simulink model "FINAL_SIMULINK_MODEL"  (R2015a)
settings: Solver=ode3  StartTime=0.0  StopTime=20  RelTol=1e-3
libraries: simulink x5, fuzblock x2
settings Model: Creator=BML  LastModifiedBy=BML
settings SolverCC: AutoInsertRateTranBlk=on

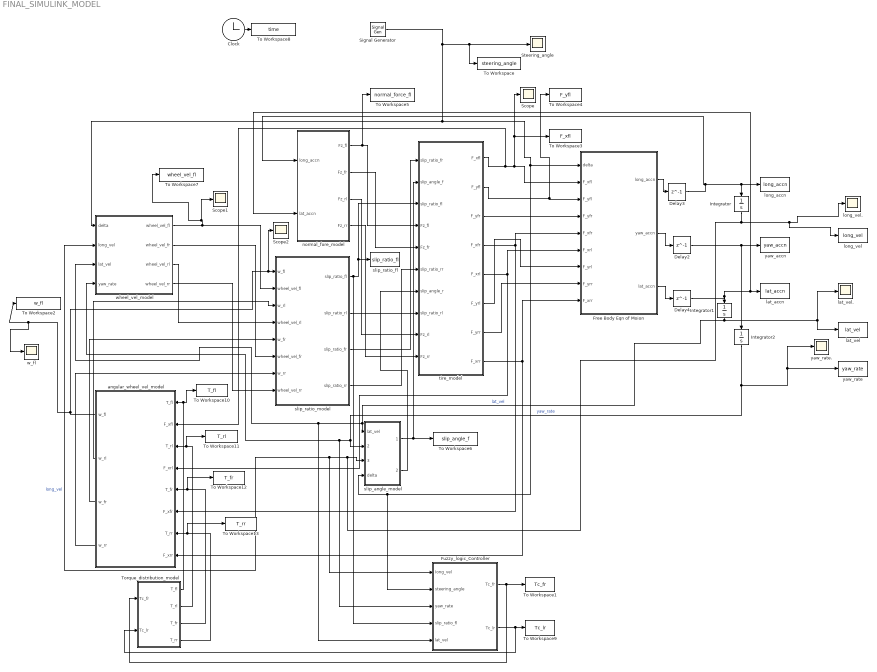
== system FINAL_SIMULINK_MODEL ==
  "           Steering_angle" : Scope
      settings: SaveName=ScopeData8
  Clock : Clock
  Delay2 : Delay  DelayLength=1  SampleTime=1
  Delay3 : Delay  DelayLength=1  SampleTime=1
  Delay4 : Delay  DelayLength=1  SampleTime=1
  Free Body Eqn of Moion : Subsystem
  Fuzzy_logic_Controller : Subsystem
  Integrator : Integrator  InitialCondition=22.22  LimitOutput=on  UpperSaturationLimit=23.22  LowerSaturationLimit=22.22
  Integrator1 : Integrator  LimitOutput=on  UpperSaturationLimit=10  LowerSaturationLimit=-10
  Integrator2 : Integrator  LimitOutput=on  UpperSaturationLimit=1  LowerSaturationLimit=-1
  Scope : Scope
      settings: SaveName=ScopeData3
  Scope1 : Scope
      settings: SaveName=ScopeData4
  Scope2 : Scope
      settings: SaveName=ScopeData6
  Signal Generator : SignalGenerator  Amplitude=2.5  Frequency=1.5  Units=rad/sec
  To Workspace : ToWorkspace  VariableName=steering_angle  SaveFormat=Timeseries  SampleTime=1
  To Workspace1 : ToWorkspace  VariableName=Tc_fr  SaveFormat=Timeseries  SampleTime=-1
  To Workspace10 : ToWorkspace  VariableName=T_fl  SaveFormat=Timeseries  SampleTime=1
  To Workspace11 : ToWorkspace  VariableName=T_rl  SaveFormat=Timeseries  SampleTime=1
  To Workspace12 : ToWorkspace  VariableName=T_fr  SaveFormat=Timeseries  SampleTime=1
  To Workspace13 : ToWorkspace  VariableName=T_rr  SaveFormat=Timeseries  SampleTime=1
  To Workspace2 : ToWorkspace  VariableName=w_fl  SaveFormat=Timeseries  SampleTime=1
  To Workspace3 : ToWorkspace  VariableName=F_xfl  SaveFormat=Timeseries  SampleTime=1
  To Workspace4 : ToWorkspace  VariableName=F_yfl  SaveFormat=Timeseries  SampleTime=1
  To Workspace5 : ToWorkspace  VariableName=normal_force_fl  SaveFormat=Timeseries  SampleTime=1
  To Workspace6 : ToWorkspace  VariableName=slip_angle_f  SaveFormat=Timeseries  SampleTime=1
  To Workspace7 : ToWorkspace  VariableName=wheel_vel_fl  SaveFormat=Timeseries  SampleTime=1
  To Workspace8 : ToWorkspace  VariableName=time  SaveFormat=Timeseries  SampleTime=1
  To Workspace9 : ToWorkspace  VariableName=Tc_lr  SaveFormat=Timeseries  SampleTime=-1
  Torque_distribution_model : Subsystem
  angular_wheel_vel_model : Subsystem
  lat_accn : ToWorkspace  VariableName=lat_accn  SaveFormat=Timeseries  SampleTime=1
  lat_vel : ToWorkspace  VariableName=lat_vel  SaveFormat=Timeseries  SampleTime=1
  lat_vel. : Scope
  long_accn : ToWorkspace  VariableName=long_accn  SaveFormat=Timeseries  SampleTime=1
  long_vel : ToWorkspace  VariableName=long_vel  SaveFormat=Timeseries  SampleTime=1
  long_vel. : Scope
  normal_fore_model : Subsystem
  slip_angle_model : Subsystem
  slip_ratio_fl : ToWorkspace  VariableName=slip_ratio_fl  SaveFormat=Timeseries  SampleTime=1
  slip_ratio_model : Subsystem
  tire_model : Subsystem
  w_fl : Scope
      settings: SaveName=ScopeData5
  wheel_vel_model : Subsystem
  yaw_accn : ToWorkspace  VariableName=yaw_accn  SaveFormat=Timeseries  SampleTime=1
  yaw_rate : ToWorkspace  VariableName=yaw_rate  SaveFormat=Timeseries  SampleTime=1
  yaw_rate. : Scope
      settings: SaveName=ScopeData2
  wires:
  slip_ratio_model/2(slip_ratio_rl) -> tire_model/8(slip_ratio_rl)
  Integrator2/1 -> slip_angle_model/2(yaw_rate), Fuzzy_logic_Controller/3(yaw_rate), wheel_vel_model/4(yaw_rate), yaw_rate./1, yaw_rate/1  "yaw_rate"
  normal_fore_model/1(Fz_fl) -> To Workspace5/1, tire_model/4(Fz_fl)
  normal_fore_model/2(Fz_fr) -> tire_model/5(Fz_fr)
  normal_fore_model/3(Fz_rl) -> tire_model/9(Fz_rl)
  normal_fore_model/4(Fz_rr) -> tire_model/10(Fz_rr)
  wheel_vel_model/3(wheel_vel_rl) -> slip_ratio_model/4(wheel_vel_rl)
  slip_ratio_model/3(slip_ratio_fr) -> tire_model/1(slip_ratio_fr)
  slip_ratio_model/4(slip_ratio_rr) -> tire_model/6(slip_ratio_rr)
  slip_angle_model/1(slip_angle_f) -> To Workspace6/1, tire_model/2("slip_angle_f  ")
  slip_angle_model/2(slip_angle_r) -> tire_model/7(slip_angle_r)
  wheel_vel_model/2(wheel_vel_fr) -> slip_ratio_model/6(wheel_vel_fr)
  wheel_vel_model/1(wheel_vel_fl) -> Scope1/1, To Workspace7/1, slip_ratio_model/2(wheel_vel_fl)
  wheel_vel_model/4(wheel_vel_rr) -> slip_ratio_model/8(wheel_vel_rr)
  Integrator/1 -> slip_angle_model/3(long_vel), Fuzzy_logic_Controller/1(Iong_vel), wheel_vel_model/2(long_vel), long_vel/1, long_vel./1  "long_vel"
  Integrator1/1 -> wheel_vel_model/3(lat_vel), Fuzzy_logic_Controller/5(lat_vel), slip_angle_model/1(lat_vel), lat_vel./1, lat_vel/1  "lat_vel"
  Free Body Eqn of Moion/2(yaw_accn) -> Delay2/1
  Free Body Eqn of Moion/1(long_accn) -> Delay3/1
  Free Body Eqn of Moion/3(lat_accn) -> Delay4/1
  angular_wheel_vel_model/4(w_rr) -> slip_ratio_model/7(w_rr)
  tire_model/3(F_yfr) -> Free Body Eqn of Moion/4(F_yfr)
  tire_model/6(F_yrl) -> Free Body Eqn of Moion/7(F_yrl)
  tire_model/7(F_yrr) -> Free Body Eqn of Moion/8(F_yrr)
  tire_model/2(F_yfl) -> To Workspace4/1, Free Body Eqn of Moion/3(F_yfl)
  Delay3/1 -> normal_fore_model/1(long_accn), Integrator/1, long_accn/1
  Delay4/1 -> normal_fore_model/2(lat_accn), lat_accn/1, Integrator1/1
  angular_wheel_vel_model/1(w_fl) -> Scope2/1, slip_ratio_model/1(w_fl), w_fl/1, To Workspace2/1
  angular_wheel_vel_model/2(w_rl) -> slip_ratio_model/3(w_rl)
  angular_wheel_vel_model/3(w_fr) -> slip_ratio_model/5(w_fr)
  Delay2/1 -> Integrator2/1, yaw_accn/1
  tire_model/1(F_xfl) -> angular_wheel_vel_model/2(F_xfl), Scope/1, To Workspace3/1, Free Body Eqn of Moion/2(F_xfl)
  tire_model/5(F_xrl) -> angular_wheel_vel_model/4(F_xrl), Free Body Eqn of Moion/6(F_xrl)
  tire_model/4(F_xfr) -> angular_wheel_vel_model/6(F_xfr), Free Body Eqn of Moion/5(F_xfr)
  tire_model/8(F_xrr) -> angular_wheel_vel_model/8(F_xrr), Free Body Eqn of Moion/9(F_xrr)
  Signal Generator/1 -> "           Steering_angle"/1, To Workspace/1, wheel_vel_model/1(delta), Fuzzy_logic_Controller/2(steering_angle), slip_angle_model/4(delta), Free Body Eqn of Moion/1(delta)
  slip_ratio_model/1(slip_ratio_fl) -> slip_ratio_fl/1, tire_model/3(slip_ratio_fl), Fuzzy_logic_Controller/4(slip_ratio_fl)
  Fuzzy_logic_Controller/1(Tc_fr) -> Torque_distribution_model/1(Tc_fr), To Workspace1/1
  Fuzzy_logic_Controller/2(Tc_lr) -> Torque_distribution_model/2(Tc_lr), To Workspace9/1
  Torque_distribution_model/1(T_fl) -> To Workspace10/1, angular_wheel_vel_model/1(T_fl)
  Torque_distribution_model/2(T_rl) -> To Workspace11/1, angular_wheel_vel_model/3(T_rl)
  Torque_distribution_model/3(T_fr) -> To Workspace12/1, angular_wheel_vel_model/5(T_fr)
  Torque_distribution_model/4(T_rr) -> To Workspace13/1, angular_wheel_vel_model/7(T_rr)
  Clock/1 -> To Workspace8/1

== system FINAL_SIMULINK_MODEL/Free Body Eqn of Moion ==
  delta : Inport
  F_xfl : Inport  Port=2
  F_yfl : Inport  Port=3
  F_yfr : Inport  Port=4
  F_xfr : Inport  Port=5
  F_xrl : Inport  Port=6
  F_yrl : Inport  Port=7
  F_yrr : Inport  Port=8
  F_xrr : Inport  Port=9
  lat_accn_model : Subsystem
  long_accn_model : Subsystem
  yaw_accn_model : Subsystem
  long_accn : Outport
  yaw_accn : Outport  Port=2
  lat_accn : Outport  Port=3
  wires:
  lat_accn_model/1(lat_accn) -> lat_accn/1
  F_yfl/1 -> long_accn_model/3(F_yfl), yaw_accn_model/3(F_yfl), lat_accn_model/3(F_yfl)
  delta/1 -> lat_accn_model/1(delta), yaw_accn_model/1(delta), long_accn_model/1(delta)
  F_xfr/1 -> long_accn_model/4(F_xfr), yaw_accn_model/4(F_xfr), lat_accn_model/4(F_xfr)
  F_yrl/1 -> yaw_accn_model/7(F_yrl), lat_accn_model/6(F_yrl)
  long_accn_model/1(long_accn) -> long_accn/1
  F_yfr/1 -> yaw_accn_model/5(F_yfr), long_accn_model/5(F_yfr), lat_accn_model/5(F_yfr)
  yaw_accn_model/1(yaw_accn) -> yaw_accn/1
  F_yrr/1 -> lat_accn_model/7(F_yrr), yaw_accn_model/9(F_yrr)
  F_xrl/1 -> long_accn_model/6(F_xrl), yaw_accn_model/6(F_xrl)
  F_xrr/1 -> long_accn_model/7(F_xrr), yaw_accn_model/8(F_xrr)
  F_xfl/1 -> long_accn_model/2(F_xfl), yaw_accn_model/2(F_xfl), lat_accn_model/2(F_xfl)

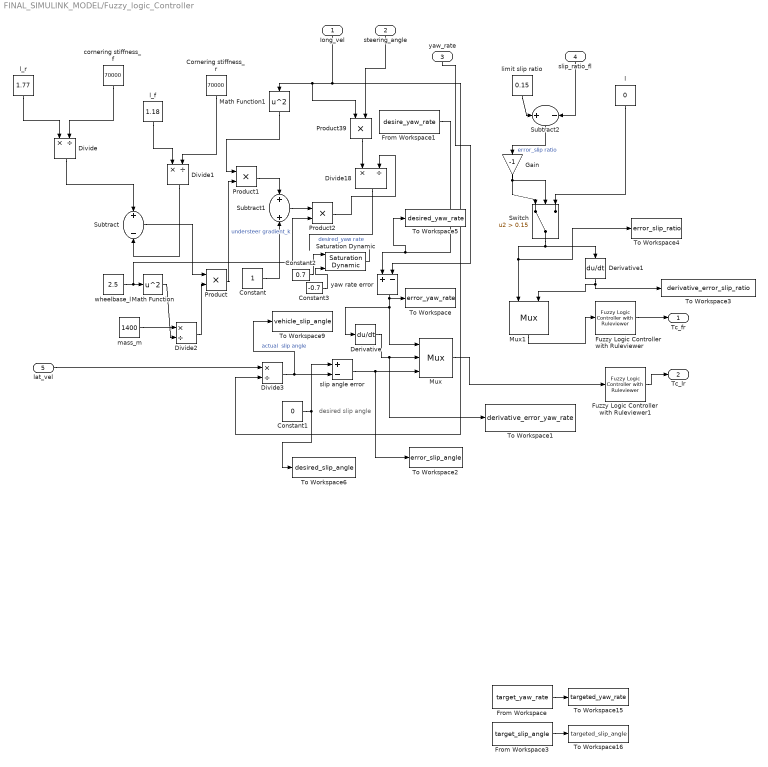
== system FINAL_SIMULINK_MODEL/Fuzzy_logic_Controller ==
  note: desired
      | slip angle
  Iong_vel : Inport
  steering_angle : Inport  Port=2
  yaw_rate : Inport  Port=3
  slip_ratio_fl : Inport  Port=4
  lat_vel : Inport  Port=5
  Constant : Constant
  Constant1 : Constant  Value=0
  Constant2 : Constant  Value=0.7
  Constant3 : Constant  Value=-0.7
  "Cornering stiffness_r " : Constant  Value=70000
  Derivative : Derivative
  Derivative1 : Derivative
  Divide{,1..3,18} (5 alike) : Product  Inputs=*/
  From Workspace : FromWorkspace  VariableName=target_yaw_rate  SampleTime=0
  From Workspace1 : FromWorkspace  VariableName=desire_yaw_rate  SampleTime=0
  From Workspace3 : FromWorkspace  VariableName=target_slip_angle  SampleTime=0
  Fuzzy Logic Controller with Ruleviewer : fuzblock/Fuzzy Logic  Controller  with Ruleviewer  fismatrix=fuzzy_slip_ratio1  Ts=2
  Fuzzy Logic Controller with Ruleviewer1 : fuzblock/Fuzzy Logic  Controller  with Ruleviewer  fismatrix=fuzzy_yaw_rate1  Ts=2
  Gain : Gain  Gain=-1
  Math Function : Math  Operator=square  SaturateOnIntegerOverflow=on
  Math Function1 : Math  Operator=square  SaturateOnIntegerOverflow=on
  Mux : Mux  Inputs=3
  Mux1 : Mux  Inputs=2
  Product{,1..2,39} (4 alike) : Product
  Saturation Dynamic : simulink/Discontinuities/Saturation Dynamic  OutMin=-0.7  OutMax=0.7  OutDataTypeStr=Inherit: Same as second input  OutDataType=fixdt(1, 16)  OutScaling=2^-10  DoSatur=off
  Subtract : Sum  Inputs=+-
  Subtract1 : Sum
  Subtract2 : Sum  Inputs=+-
  Switch : Switch  Criteria=u2 > Threshold  Threshold=0.15
  To Workspace : ToWorkspace  VariableName=error_yaw_rate  SaveFormat=Timeseries  SampleTime=1
  To Workspace1 : ToWorkspace  VariableName=derivative_error_yaw_rate  SaveFormat=Timeseries  SampleTime=1
  To Workspace15 : ToWorkspace  VariableName=targeted_yaw_rate  SaveFormat=Timeseries  SampleTime=1
  To Workspace16 : ToWorkspace  VariableName=targeted_slip_angle  SaveFormat=Timeseries  SampleTime=1
  To Workspace2 : ToWorkspace  VariableName=error_slip_angle  SaveFormat=Timeseries  SampleTime=1
  To Workspace3 : ToWorkspace  VariableName=derivative_error_slip_ratio  SaveFormat=Timeseries  SampleTime=1
  To Workspace4 : ToWorkspace  VariableName=error_slip_ratio  SaveFormat=Timeseries  SampleTime=1
  To Workspace5 : ToWorkspace  VariableName=desired_yaw_rate  SaveFormat=Timeseries  SampleTime=1
  To Workspace6 : ToWorkspace  VariableName=desired_slip_angle  SaveFormat=Timeseries  SampleTime=1
  To Workspace9 : ToWorkspace  VariableName=vehicle_slip_angle  SaveFormat=Timeseries  SampleTime=1
  "cornering stiffness_f " : Constant  Value=70000
  l : Constant  Value=0
  "l_f " : Constant  Value=1.18
  "l_r " : Constant  Value=1.77
  limit slip ratio : Constant  Value=0.15
  mass_m : Constant  Value=1400
  "slip angle error  " : Sum  Inputs=+-
  wheelbase_l : Constant  Value=2.5
  "yaw rate error   " : Sum  Inputs=+-
  Tc_fr : Outport
  Tc_lr : Outport  Port=2
  wires:
  Fuzzy Logic Controller with Ruleviewer/1 -> Tc_fr/1
  Divide/1 -> Subtract/1
  Subtract/1 -> Product/1
  Product/1 -> Product1/2  "understeer gradient_k"
  Constant/1 -> Subtract1/2
  Product39/1 -> Divide18/1
  Product2/1 -> Divide18/2
  steering_angle/1 -> Product39/2
  Math Function1/1 -> Product1/1
  Subtract1/1 -> Product2/1
  lat_vel/1 -> Divide3/1
  "l_r "/1 -> Divide/1
  Divide1/1 -> Subtract/2
  "Cornering stiffness_r "/1 -> Divide1/2
  wheelbase_l/1 -> Product2/2, Math Function/1
  mass_m/1 -> Divide2/1
  Math Function/1 -> Divide2/2
  Divide2/1 -> Product/2
  "l_f "/1 -> Divide1/1
  "cornering stiffness_f "/1 -> Divide/2
  Product1/1 -> Subtract1/1
  Switch/1 -> Mux1/1, To Workspace4/1, Derivative1/1
  yaw_rate/1 -> "yaw rate error   "/2
  Divide18/1 -> ?  "desired_yaw rate"
  Subtract2/1 -> Gain/1  "error_slip ratio"
  limit slip ratio/1 -> Subtract2/1
  Derivative/1 -> To Workspace1/1, Mux/2
  Mux/1 -> Fuzzy Logic Controller with Ruleviewer1/1
  slip_ratio_fl/1 -> Subtract2/2
  Divide3/1 -> To Workspace9/1, "slip angle error  "/2  "actual  slip angle"
  "slip angle error  "/1 -> To Workspace2/1, Mux/3
  Derivative1/1 -> Mux1/2, To Workspace3/1
  Mux1/1 -> Fuzzy Logic Controller with Ruleviewer/1
  Fuzzy Logic Controller with Ruleviewer1/1 -> Tc_lr/1
  "yaw rate error   "/1 -> To Workspace/1, Mux/1, Derivative/1
  Constant1/1 -> "slip angle error  "/1, To Workspace6/1
  Iong_vel/1 -> Divide3/2, Math Function1/1, Product39/1
  l/1 -> Switch/3
  Gain/1 -> Switch/1, Switch/2
  Constant2/1 -> Saturation Dynamic/1
  Constant3/1 -> Saturation Dynamic/3
  Saturation Dynamic/1 -> ?
  From Workspace1/1 -> To Workspace5/1, "yaw rate error   "/1
  From Workspace/1 -> To Workspace15/1
  From Workspace3/1 -> To Workspace16/1

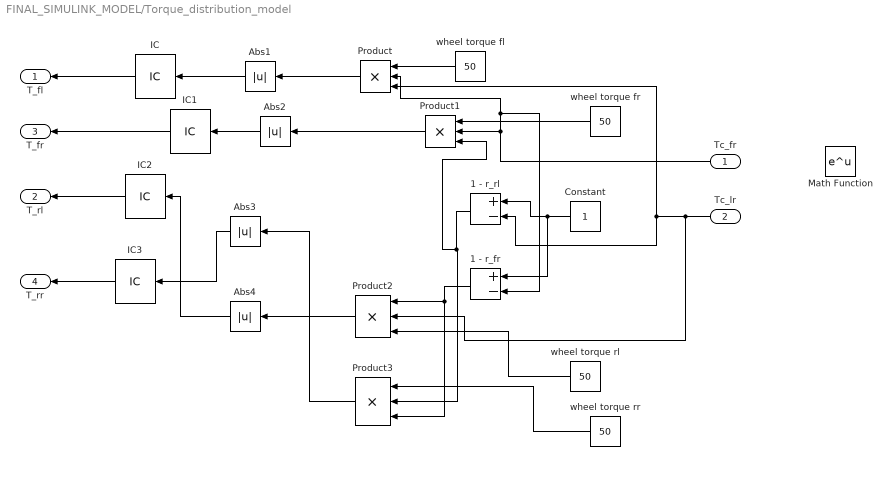
== system FINAL_SIMULINK_MODEL/Torque_distribution_model ==
  Tc_fr : Inport
  Tc_lr : Inport  Port=2
  1 - r_fr : Sum  Inputs=+-
  1 - r_rl : Sum  Inputs=+-
  Abs{1..4} (4 alike) : Abs
  Constant : Constant
  IC{,1..3} (4 alike) : InitialCondition  Value=50
  Math Function : Math  SaturateOnIntegerOverflow=on
  Product{,1..3} (4 alike) : Product  Inputs=3
  wheel torque fl : Constant  Value=50
  wheel torque fr : Constant  Value=50
  wheel torque rl : Constant  Value=50
  wheel torque rr : Constant  Value=50
  T_fl : Outport
  T_rl : Outport  Port=2
  T_fr : Outport  Port=3
  T_rr : Outport  Port=4
  wires:
  1 - r_rl/1 -> Product3/2, Product1/3
  Constant/1 -> 1 - r_fr/1, 1 - r_rl/1
  1 - r_fr/1 -> Product3/3, Product2/1
  wheel torque fl/1 -> Product/1
  Tc_fr/1 -> Product/2, 1 - r_fr/2, Product1/2
  Product1/1 -> Abs2/1
  Product3/1 -> Abs3/1
  Product2/1 -> Abs4/1
  Product/1 -> Abs1/1
  Tc_lr/1 -> Product2/2, 1 - r_rl/2, Product/3
  wheel torque fr/1 -> Product1/1
  wheel torque rl/1 -> Product2/3
  wheel torque rr/1 -> Product3/1
  Abs1/1 -> IC/1
  Abs2/1 -> IC1/1
  Abs3/1 -> IC3/1
  Abs4/1 -> IC2/1
  IC/1 -> T_fl/1
  IC1/1 -> T_fr/1
  IC2/1 -> T_rl/1
  IC3/1 -> T_rr/1

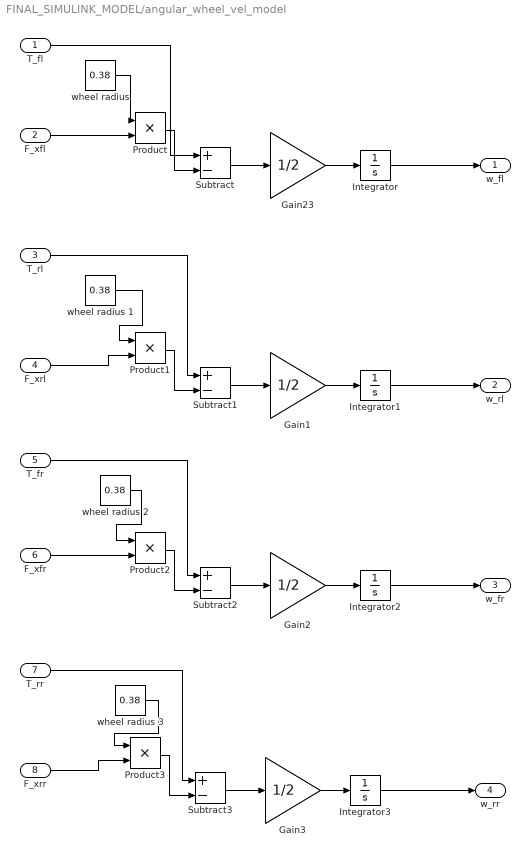
== system FINAL_SIMULINK_MODEL/angular_wheel_vel_model ==
  T_fl : Inport
  F_xfl : Inport  Port=2
  T_rl : Inport  Port=3
  F_xrl : Inport  Port=4
  T_fr : Inport  Port=5
  F_xfr : Inport  Port=6
  T_rr : Inport  Port=7
  F_xrr : Inport  Port=8
  Gain{1..3,23} (4 alike) : Gain  Gain=1/2
  Integrator{,1..3} (4 alike) : Integrator  InitialCondition=58.5  LimitOutput=on  UpperSaturationLimit=70  LowerSaturationLimit=57
  Product{,1..3} (4 alike) : Product
  Subtract{,1..3} (4 alike) : Sum  Inputs=+-
  wheel radius {,1..3} (4 alike) : Constant  Value=0.38
  w_fl : Outport
  w_rl : Outport  Port=2
  w_fr : Outport  Port=3
  w_rr : Outport  Port=4
  wires:
  Gain23/1 -> Integrator/1
  F_xfl/1 -> Product/2
  Product/1 -> Subtract/2
  wheel radius 1/1 -> Product1/1
  T_rl/1 -> Subtract1/1
  T_fl/1 -> Subtract/1
  Subtract/1 -> Gain23/1
  F_xrl/1 -> Product1/2
  "wheel radius "/1 -> Product/1
  Subtract2/1 -> Gain2/1
  wheel radius 2/1 -> Product2/1
  Product1/1 -> Subtract1/2
  F_xrr/1 -> Product3/2
  T_rr/1 -> Subtract3/1
  Gain3/1 -> Integrator3/1
  Subtract1/1 -> Gain1/1
  Gain1/1 -> Integrator1/1
  Gain2/1 -> Integrator2/1
  Subtract3/1 -> Gain3/1
  wheel radius 3/1 -> Product3/1
  F_xfr/1 -> Product2/2
  Product3/1 -> Subtract3/2
  T_fr/1 -> Subtract2/1
  Product2/1 -> Subtract2/2
  Integrator/1 -> w_fl/1
  Integrator1/1 -> w_rl/1
  Integrator2/1 -> w_fr/1
  Integrator3/1 -> w_rr/1

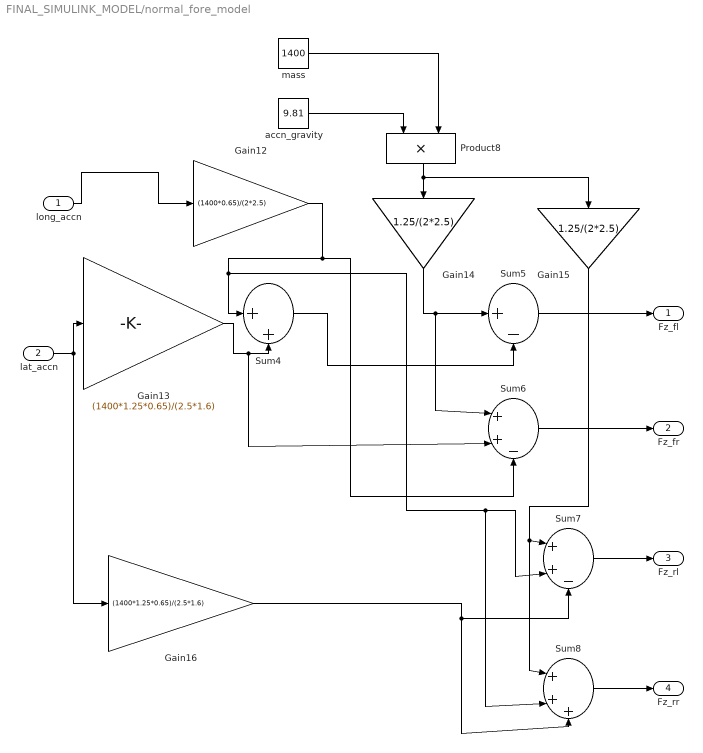
== system FINAL_SIMULINK_MODEL/normal_fore_model ==
  long_accn : Inport
  lat_accn : Inport  Port=2
  Gain12 : Gain  Gain=(1400*0.65)/(2*2.5)
  Gain13 : Gain  Gain=(1400*1.25*0.65)/(2.5*1.6)
  Gain14 : Gain  Gain=1.25/(2*2.5)
  Gain15 : Gain  Gain=1.25/(2*2.5)
  Gain16 : Gain  Gain=(1400*1.25*0.65)/(2.5*1.6)
  Product8 : Product
  Sum4 : Sum  Inputs=|++
  Sum5 : Sum  Inputs=|+-
  Sum6 : Sum  Inputs=|++-
  Sum7 : Sum  Inputs=|++-
  Sum8 : Sum  Inputs=|+++
  "accn_gravity " : Constant  Value=9.81
  mass : Constant  Value=1400
  Fz_fl : Outport
  Fz_fr : Outport  Port=2
  Fz_rl : Outport  Port=3
  Fz_rr : Outport  Port=4
  wires:
  Gain12/1 -> Sum4/1, Sum8/2, Sum7/2, Sum6/3
  Gain15/1 -> Sum8/1, Sum7/1
  Gain16/1 -> Sum8/3, Sum7/3
  Sum7/1 -> Fz_rl/1
  lat_accn/1 -> Gain13/1, Gain16/1
  Gain13/1 -> Sum6/2, Sum4/2
  Sum5/1 -> Fz_fl/1
  Sum6/1 -> Fz_fr/1
  Sum4/1 -> Sum5/2
  long_accn/1 -> Gain12/1
  mass/1 -> Product8/2
  Gain14/1 -> Sum5/1, Sum6/1
  Sum8/1 -> Fz_rr/1
  Product8/1 -> Gain14/1, Gain15/1
  "accn_gravity "/1 -> Product8/1

== system FINAL_SIMULINK_MODEL/slip_angle_model ==
  lat_vel : Inport
  yaw_rate : Inport  Port=2
  long_vel : Inport  Port=3
  delta : Inport  Port=4
  Divide4 : Product  Inputs=*/
  Divide5 : Product  Inputs=*/
  Product : Product
  Product1 : Product
  Sum4 : Sum  Inputs=|++
  Sum5 : Sum  Inputs=|+-
  Sum6 : Sum  Inputs=|+-
  l_f : Constant  Value=1.25
  l_r : Constant  Value=1.25
  slip_angle_f : Outport
  slip_angle_r : Outport  Port=2
  wires:
  yaw_rate/1 -> Product1/2, Product/2
  long_vel/1 -> Divide5/2, Divide4/2
  l_f/1 -> Product/1
  lat_vel/1 -> Sum6/2, Sum4/1
  Divide4/1 -> Sum5/2
  Product/1 -> Sum4/2
  Sum4/1 -> Divide4/1
  Divide5/1 -> slip_angle_r/1
  delta/1 -> Sum5/1
  Sum5/1 -> slip_angle_f/1
  Product1/1 -> Sum6/1
  l_r/1 -> Product1/1
  Sum6/1 -> Divide5/1

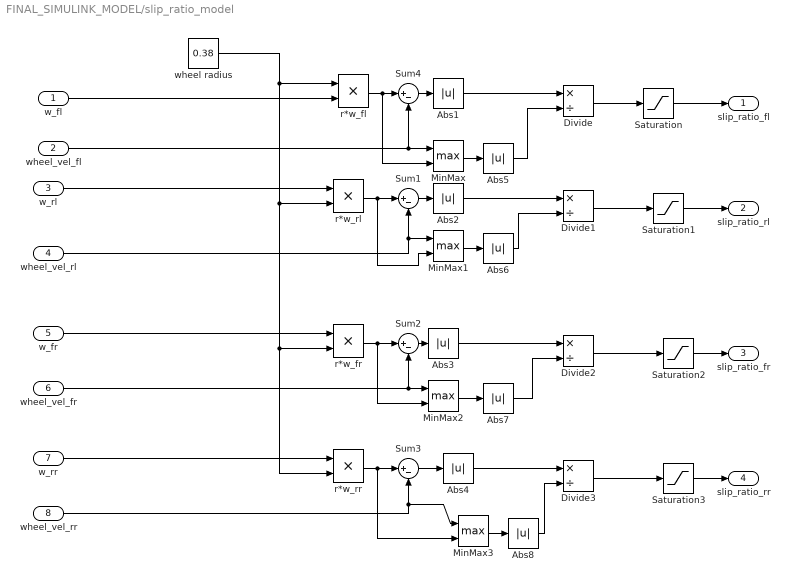
== system FINAL_SIMULINK_MODEL/slip_ratio_model ==
  w_fl : Inport
  wheel_vel_fl : Inport  Port=2
  w_rl : Inport  Port=3
  wheel_vel_rl : Inport  Port=4
  w_fr : Inport  Port=5
  wheel_vel_fr : Inport  Port=6
  w_rr : Inport  Port=7
  wheel_vel_rr : Inport  Port=8
  Abs{1..8} (8 alike) : Abs
  Divide{,1..3} (4 alike) : Product  Inputs=*/
  MinMax{,1..3} (4 alike) : MinMax  Function=max  Inputs=2
  Saturation{,1..3} (4 alike) : Saturate  UpperLimit=1  LowerLimit=0
  Sum{1..4} (4 alike) : Sum  Inputs=|+-
  r*w_fl : Product  Inputs=**
  r*w_fr : Product  Inputs=**
  r*w_rl : Product  Inputs=**
  r*w_rr : Product  Inputs=**
  wheel radius : Constant  Value=0.38
  slip_ratio_fl : Outport
  slip_ratio_rl : Outport  Port=2
  slip_ratio_fr : Outport  Port=3
  slip_ratio_rr : Outport  Port=4
  wires:
  w_fl/1 -> r*w_fl/2
  r*w_fl/1 -> MinMax/2, Sum4/1
  wheel radius/1 -> r*w_fl/1, r*w_rl/2, r*w_rr/2, r*w_fr/2
  wheel_vel_fl/1 -> MinMax/1, Sum4/2
  Sum4/1 -> Abs1/1
  Abs1/1 -> Divide/1
  MinMax/1 -> Abs5/1
  r*w_rl/1 -> MinMax1/2, Sum1/1
  wheel_vel_rl/1 -> Sum1/2, MinMax1/1
  Sum1/1 -> Abs2/1
  Abs2/1 -> Divide1/1
  MinMax1/1 -> Abs6/1
  w_rl/1 -> r*w_rl/1
  r*w_fr/1 -> MinMax2/2, Sum2/1
  wheel_vel_fr/1 -> Sum2/2, MinMax2/1
  Sum2/1 -> Abs3/1
  Abs3/1 -> Divide2/1
  MinMax2/1 -> Abs7/1
  w_fr/1 -> r*w_fr/1
  r*w_rr/1 -> MinMax3/2, Sum3/1
  wheel_vel_rr/1 -> MinMax3/1, Sum3/2
  Sum3/1 -> Abs4/1
  Abs4/1 -> Divide3/1
  MinMax3/1 -> Abs8/1
  w_rr/1 -> r*w_rr/1
  Divide/1 -> Saturation/1
  Divide1/1 -> Saturation1/1
  Divide2/1 -> Saturation2/1
  Divide3/1 -> Saturation3/1
  Abs5/1 -> Divide/2
  Abs6/1 -> Divide1/2
  Abs7/1 -> Divide2/2
  Abs8/1 -> Divide3/2
  Saturation/1 -> slip_ratio_fl/1
  Saturation1/1 -> slip_ratio_rl/1
  Saturation2/1 -> slip_ratio_fr/1
  Saturation3/1 -> slip_ratio_rr/1

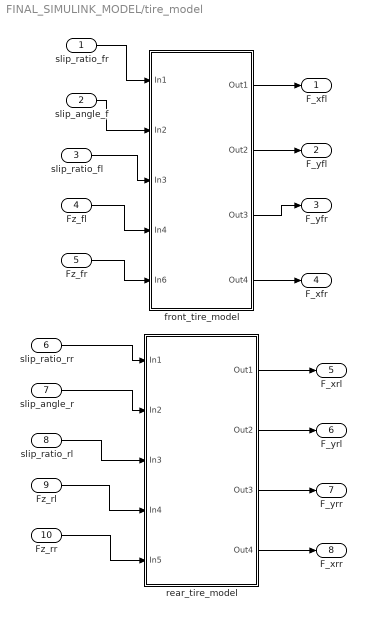
== system FINAL_SIMULINK_MODEL/tire_model ==
  slip_ratio_fr : Inport
  "slip_angle_f  " : Inport  Port=2
  slip_ratio_fl : Inport  Port=3
  Fz_fl : Inport  Port=4
  Fz_fr : Inport  Port=5
  slip_ratio_rr : Inport  Port=6
  slip_angle_r : Inport  Port=7
  slip_ratio_rl : Inport  Port=8
  Fz_rl : Inport  Port=9
  Fz_rr : Inport  Port=10
  front_tire_model : Subsystem
  rear_tire_model : Subsystem
  F_xfl : Outport
  F_yfl : Outport  Port=2
  F_yfr : Outport  Port=3
  F_xfr : Outport  Port=4
  F_xrl : Outport  Port=5
  F_yrl : Outport  Port=6
  F_yrr : Outport  Port=7
  F_xrr : Outport  Port=8
  wires:
  slip_ratio_rr/1 -> rear_tire_model/1(In1)
  slip_angle_r/1 -> rear_tire_model/2(In2)
  rear_tire_model/3(Out3) -> F_yrr/1
  slip_ratio_rl/1 -> rear_tire_model/3(In3)
  rear_tire_model/2(Out2) -> F_yrl/1
  Fz_rr/1 -> rear_tire_model/5(In5)
  rear_tire_model/1(Out1) -> F_xrl/1
  rear_tire_model/4(Out4) -> F_xrr/1
  Fz_rl/1 -> rear_tire_model/4(In4)
  "slip_angle_f  "/1 -> front_tire_model/2(In2)
  slip_ratio_fr/1 -> front_tire_model/1(In1)
  slip_ratio_fl/1 -> front_tire_model/3(In3)
  Fz_fr/1 -> front_tire_model/5(In6)
  front_tire_model/1(Out1) -> F_xfl/1
  front_tire_model/3(Out3) -> F_yfr/1
  front_tire_model/2(Out2) -> F_yfl/1
  Fz_fl/1 -> front_tire_model/4(In4)
  front_tire_model/4(Out4) -> F_xfr/1

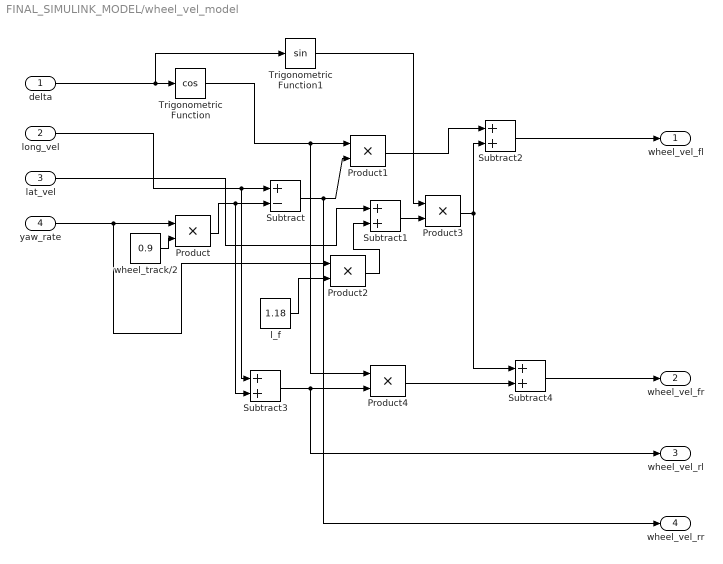
== system FINAL_SIMULINK_MODEL/wheel_vel_model ==
  delta : Inport
  long_vel : Inport  Port=2
  lat_vel : Inport  Port=3
  yaw_rate : Inport  Port=4
  Product{,1..4} (5 alike) : Product
  Subtract : Sum  Inputs=+-
  Subtract{1..4} (4 alike) : Sum
  Trigonometric Function : Trigonometry  Operator=cos
  Trigonometric Function1 : Trigonometry
  l_f : Constant  Value=1.18
  wheel_track/2 : Constant  Value=0.9
  wheel_vel_fl : Outport
  wheel_vel_fr : Outport  Port=2
  wheel_vel_rl : Outport  Port=3
  wheel_vel_rr : Outport  Port=4
  wires:
  long_vel/1 -> Subtract3/1, Subtract/1
  l_f/1 -> Product2/2
  Subtract3/1 -> wheel_vel_rl/1, Product4/2
  Trigonometric Function/1 -> Product4/1, Product1/1
  Subtract1/1 -> Product3/2
  Subtract/1 -> wheel_vel_rr/1, Product1/2
  Product4/1 -> Subtract4/2
  Subtract4/1 -> wheel_vel_fr/1
  lat_vel/1 -> Subtract1/1
  Product/1 -> Subtract3/2, Subtract/2
  Product2/1 -> Subtract1/2
  Product1/1 -> Subtract2/1
  yaw_rate/1 -> Product/1, Product2/1
  wheel_track/2/1 -> Product/2
  Trigonometric Function1/1 -> Product3/1
  Subtract2/1 -> wheel_vel_fl/1
  delta/1 -> Trigonometric Function1/1, Trigonometric Function/1
  Product3/1 -> Subtract2/2, Subtract4/1

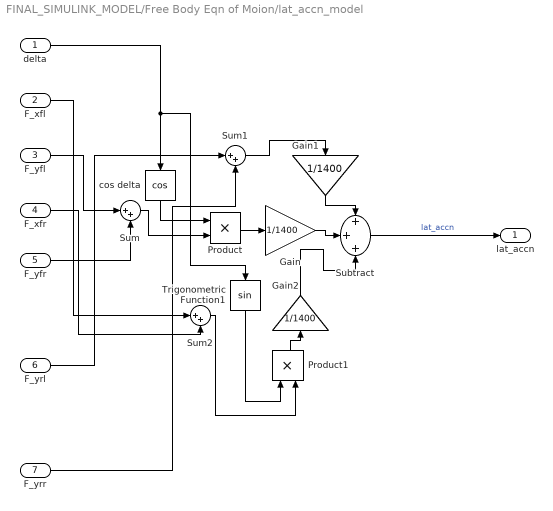
== system FINAL_SIMULINK_MODEL/Free Body Eqn of Moion/lat_accn_model ==
  delta : Inport
  F_xfl : Inport  Port=2
  F_yfl : Inport  Port=3
  F_xfr : Inport  Port=4
  F_yfr : Inport  Port=5
  F_yrl : Inport  Port=6
  F_yrr : Inport  Port=7
  Gain : Gain  Gain=1/1400
  Gain1 : Gain  Gain=1/1400
  Gain2 : Gain  Gain=1/1400
  Product : Product
  Product1 : Product
  Subtract : Sum  Inputs=+++
  Sum : Sum  Inputs=|++
  Sum1 : Sum  Inputs=|++
  Sum2 : Sum  Inputs=|++
  Trigonometric Function1 : Trigonometry
  cos delta : Trigonometry  Operator=cos
  lat_accn : Outport
  wires:
  Gain/1 -> Subtract/2
  cos delta/1 -> Product/1
  Sum/1 -> Product/2
  Gain1/1 -> Subtract/1
  Sum1/1 -> Gain1/1
  Product/1 -> Gain/1
  delta/1 -> Trigonometric Function1/1, cos delta/1
  Trigonometric Function1/1 -> Product1/1
  Sum2/1 -> Product1/2
  Subtract/1 -> lat_accn/1  "lat_accn"
  Product1/1 -> Gain2/1
  F_xfr/1 -> Sum2/2
  F_xfl/1 -> Sum2/1
  Gain2/1 -> Subtract/3
  F_yfr/1 -> Sum/2
  F_yrl/1 -> Sum1/1
  F_yfl/1 -> Sum/1
  F_yrr/1 -> Sum1/2

== system FINAL_SIMULINK_MODEL/Free Body Eqn of Moion/long_accn_model ==
  delta : Inport
  F_xfl : Inport  Port=2
  F_yfl : Inport  Port=3
  F_xfr : Inport  Port=4
  F_yfr : Inport  Port=5
  F_xrl : Inport  Port=6
  F_xrr : Inport  Port=7
  Gain : Gain  Gain=1/1400
  Gain1 : Gain  Gain=1/1400
  Gain2 : Gain  Gain=1/1400
  Product : Product
  Product1 : Product
  Subtract : Sum  Inputs=++-
  Sum : Sum  Inputs=|++
  Sum1 : Sum  Inputs=|++
  Sum2 : Sum  Inputs=|++
  Trigonometric Function1 : Trigonometry
  cos delta : Trigonometry  Operator=cos
  long_accn : Outport
  wires:
  Gain/1 -> Subtract/2
  cos delta/1 -> Product/1
  Sum/1 -> Product/2
  Product/1 -> Gain/1
  Gain1/1 -> Subtract/1
  F_xrr/1 -> Sum1/2
  Sum1/1 -> Gain1/1
  F_xfr/1 -> Sum/2
  F_xrl/1 -> Sum1/1
  F_xfl/1 -> Sum/1
  F_yfl/1 -> Sum2/1
  F_yfr/1 -> Sum2/2
  Product1/1 -> Gain2/1
  delta/1 -> Trigonometric Function1/1, cos delta/1
  Trigonometric Function1/1 -> Product1/1
  Subtract/1 -> long_accn/1  "long_accn"
  Sum2/1 -> Product1/2
  Gain2/1 -> Subtract/3

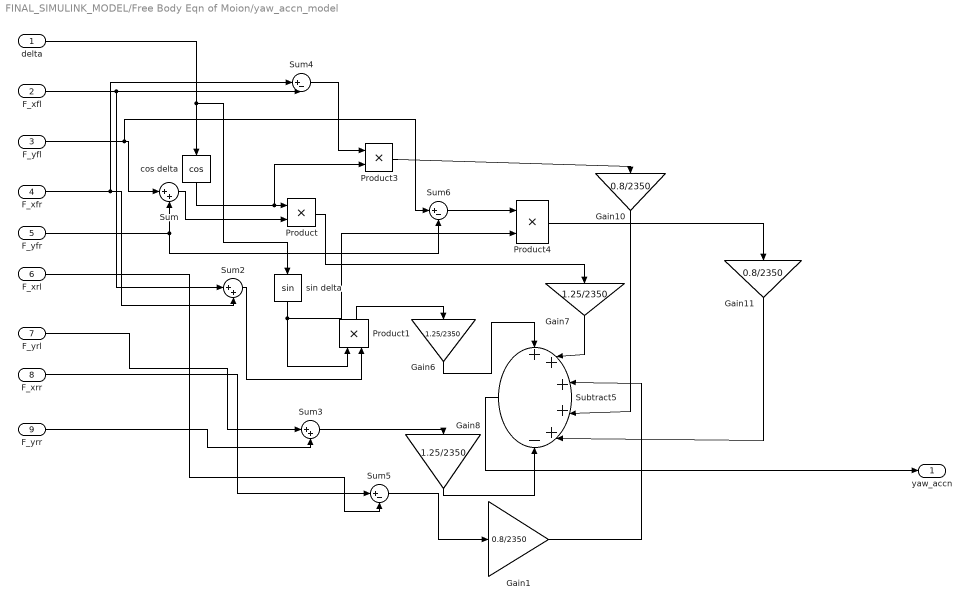
== system FINAL_SIMULINK_MODEL/Free Body Eqn of Moion/yaw_accn_model ==
  delta : Inport
  F_xfl : Inport  Port=2
  F_yfl : Inport  Port=3
  F_xfr : Inport  Port=4
  F_yfr : Inport  Port=5
  F_xrl : Inport  Port=6
  F_yrl : Inport  Port=7
  F_xrr : Inport  Port=8
  F_yrr : Inport  Port=9
  Gain1 : Gain  Gain=0.8/2350
  Gain10 : Gain  Gain=0.8/2350
  Gain11 : Gain  Gain=0.8/2350
  Gain6 : Gain  Gain=1.25/2350
  Gain7 : Gain  Gain=1.25/2350
  Gain8 : Gain  Gain=1.25/2350
  Product{,1,3..4} (4 alike) : Product
  Subtract5 : Sum  Inputs=+++++-
  Sum : Sum  Inputs=|++
  Sum2 : Sum  Inputs=|++
  Sum3 : Sum  Inputs=|++
  Sum4 : Sum  Inputs=|+-
  Sum5 : Sum  Inputs=|+-
  Sum6 : Sum  Inputs=|+-
  cos delta : Trigonometry  Operator=cos
  "sin delta " : Trigonometry
  yaw_accn : Outport
  wires:
  Sum4/1 -> Product3/1
  delta/1 -> "sin delta "/1, cos delta/1
  F_yrl/1 -> Sum3/1
  Product3/1 -> Gain10/1
  Gain10/1 -> Subtract5/4
  F_xrr/1 -> Sum5/1
  F_yfl/1 -> Sum6/1, Sum/1
  Gain11/1 -> Subtract5/5
  F_yrr/1 -> Sum3/2
  F_xrl/1 -> Sum5/2
  "sin delta "/1 -> Product4/2, Product1/1
  cos delta/1 -> Product3/2, Product/1
  Gain7/1 -> Subtract5/2
  F_yfr/1 -> Sum6/2, Sum/2
  Gain6/1 -> Subtract5/1
  Gain8/1 -> Subtract5/6
  Product/1 -> Gain7/1
  F_xfl/1 -> Sum2/1, Sum4/2
  Product1/1 -> Gain6/1
  Sum3/1 -> Gain8/1
  Sum/1 -> Product/2
  Sum2/1 -> Product1/2
  F_xfr/1 -> Sum4/1, Sum2/2
  Sum6/1 -> Product4/1
  Subtract5/1 -> yaw_accn/1
  Sum5/1 -> Gain1/1
  Gain1/1 -> Subtract5/3
  Product4/1 -> Gain11/1

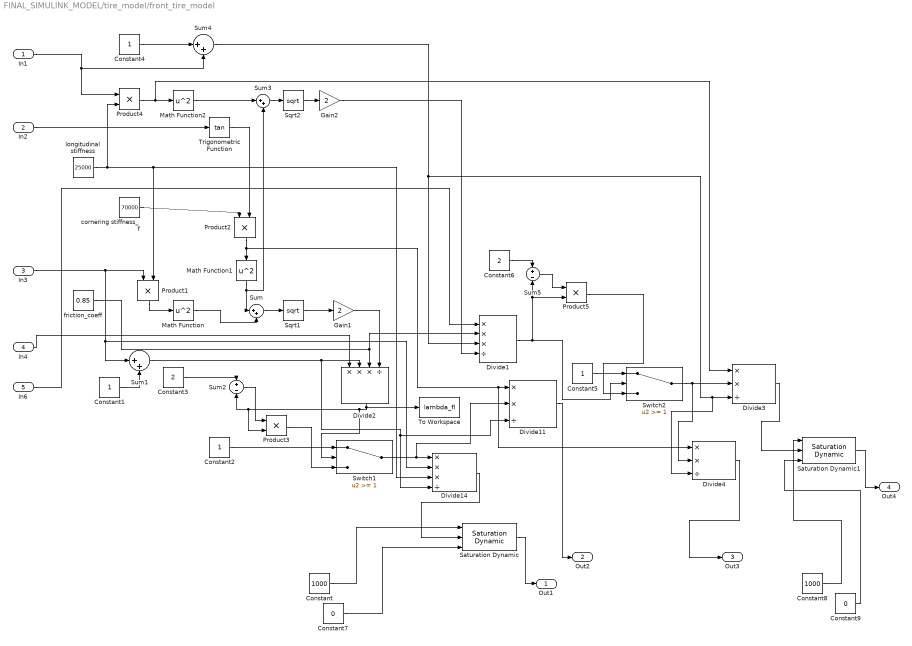
== system FINAL_SIMULINK_MODEL/tire_model/front_tire_model ==
  In1 : Inport
  In2 : Inport  Port=2
  In3 : Inport  Port=3
  In4 : Inport  Port=4
  In6 : Inport  Port=5
  Constant : Constant  Value=1000
  Constant{1..2,4..5} (4 alike) : Constant
  Constant3 : Constant  Value=2
  Constant6 : Constant  Value=2
  Constant7 : Constant  Value=0
  Constant8 : Constant  Value=1000
  Constant9 : Constant  Value=0
  Divide1 : Product  Inputs=***/
  Divide11 : Product  Inputs=**/
  Divide14 : Product  Inputs=***/
  Divide2 : Product  Inputs=***/
  Divide3 : Product  Inputs=**/
  Divide4 : Product  Inputs=**/
  Gain1 : Gain  Gain=2
  Gain2 : Gain  Gain=2
  Math Function : Math  Operator=square  SaturateOnIntegerOverflow=on
  Math Function1 : Math  Operator=square  SaturateOnIntegerOverflow=on
  Math Function2 : Math  Operator=square  SaturateOnIntegerOverflow=on
  Product{1..5} (5 alike) : Product
  Saturation Dynamic : simulink/Discontinuities/Saturation Dynamic  OutMin=0  OutMax=1000  OutDataTypeStr=Inherit: Same as second input  OutDataType=fixdt(1, 16)  OutScaling=2^-10  DoSatur=off
  Saturation Dynamic1 : simulink/Discontinuities/Saturation Dynamic  OutMin=0  OutMax=1000  OutDataTypeStr=Inherit: Same as second input  OutDataType=fixdt(1, 16)  OutScaling=2^-10  DoSatur=off
  Sqrt1 : Sqrt  SaturateOnIntegerOverflow=on
  Sqrt2 : Sqrt  SaturateOnIntegerOverflow=on
  Sum{,1,3..4} (4 alike) : Sum  Inputs=|++
  Sum2 : Sum  Inputs=+-
  Sum5 : Sum  Inputs=+-
  Switch1 : Switch  Threshold=1
  Switch2 : Switch  Threshold=1
  To Workspace : ToWorkspace  VariableName=lambda_fl  SaveFormat=Timeseries  SampleTime=-1
  Trigonometric Function : Trigonometry  Operator=tan
  cornering stiffness_f : Constant  Value=70000
  friction_coeff : Constant  Value=0.85
  longitudinal stiffness : Constant  Value=25000
  Out1 : Outport
  Out2 : Outport  Port=2
  Out3 : Outport  Port=3
  Out4 : Outport  Port=4
  wires:
  Math Function/1 -> Sum/2
  Constant1/1 -> Sum1/2
  Gain1/1 -> Divide2/4
  Trigonometric Function/1 -> Product2/2
  In3/1 -> Divide14/2, Sum1/1, Product1/1
  Sum/1 -> Sqrt1/1
  friction_coeff/1 -> Divide1/2, Divide2/3
  Sqrt1/1 -> Gain1/1
  In4/1 -> Divide2/1
  Product3/1 -> Switch1/3
  Gain2/1 -> Divide1/4
  Math Function1/1 -> Sum3/2, Sum/1
  Sum5/1 -> Product5/1
  Product2/1 -> Divide4/1, Divide11/1, Math Function1/1
  Constant5/1 -> Switch2/1
  cornering stiffness_f/1 -> Product2/1
  Switch2/1 -> Divide4/2, Divide3/2
  In6/1 -> Divide1/1
  Sum4/1 -> Divide4/3, Divide3/3, Divide1/3
  Constant2/1 -> Switch1/1
  Sum1/1 -> Divide11/3, Divide14/4, Divide2/2
  In1/1 -> Sum4/2, Product4/1
  Switch1/1 -> Divide11/2, Divide14/1
  Constant4/1 -> Sum4/1
  longitudinal stiffness/1 -> Product4/2, Product1/2, Divide14/3
  Sum3/1 -> Sqrt2/1
  Math Function2/1 -> Sum3/1
  Constant6/1 -> Sum5/1
  Sqrt2/1 -> Gain2/1
  Product4/1 -> Divide3/1, Math Function2/1
  Sum2/1 -> Product3/1
  Divide1/1 -> Switch2/2, Sum5/2, Product5/2
  Constant3/1 -> Sum2/1
  Product1/1 -> Math Function/1
  In2/1 -> Trigonometric Function/1
  Divide2/1 -> Switch1/2, Product3/2, Sum2/2, To Workspace/1
  Product5/1 -> Switch2/3
  Divide11/1 -> Out2/1
  Divide4/1 -> Out3/1
  Divide14/1 -> Saturation Dynamic/2
  Constant/1 -> Saturation Dynamic/1
  Constant7/1 -> Saturation Dynamic/3
  Saturation Dynamic/1 -> Out1/1
  Saturation Dynamic1/1 -> Out4/1
  Divide3/1 -> Saturation Dynamic1/2
  Constant8/1 -> Saturation Dynamic1/1
  Constant9/1 -> Saturation Dynamic1/3

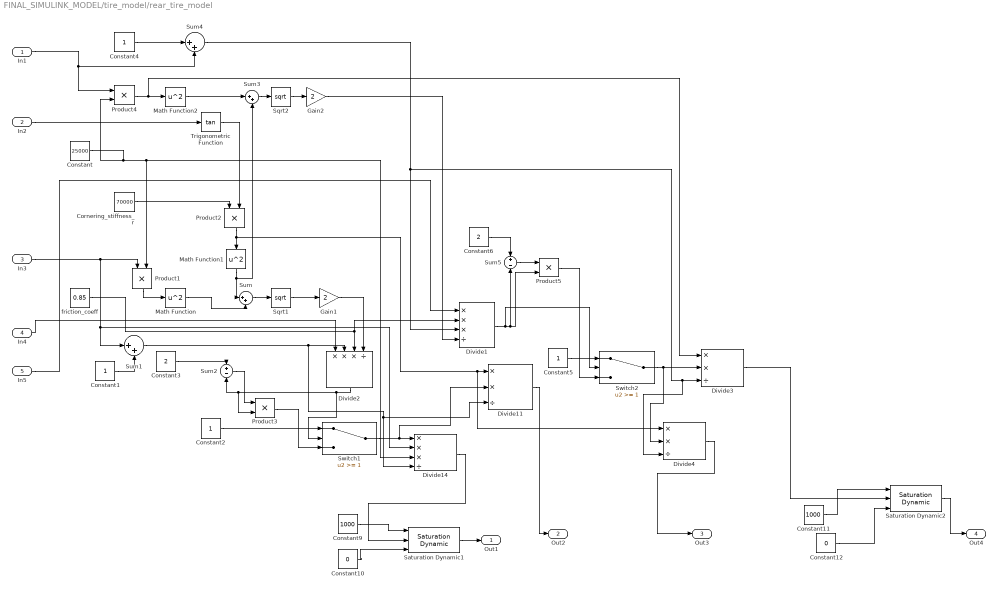
== system FINAL_SIMULINK_MODEL/tire_model/rear_tire_model ==
  In1 : Inport
  In2 : Inport  Port=2
  In3 : Inport  Port=3
  In4 : Inport  Port=4
  In5 : Inport  Port=5
  Constant : Constant  Value=25000
  Constant{1..2,4..5} (4 alike) : Constant
  Constant10 : Constant  Value=0
  Constant11 : Constant  Value=1000
  Constant12 : Constant  Value=0
  Constant3 : Constant  Value=2
  Constant6 : Constant  Value=2
  Constant9 : Constant  Value=1000
  "Cornering_stiffness_r          " : Constant  Value=70000
  Divide1 : Product  Inputs=***/
  Divide11 : Product  Inputs=**/
  Divide14 : Product  Inputs=***/
  Divide2 : Product  Inputs=***/
  Divide3 : Product  Inputs=**/
  Divide4 : Product  Inputs=**/
  Gain1 : Gain  Gain=2
  Gain2 : Gain  Gain=2
  Math Function : Math  Operator=square  SaturateOnIntegerOverflow=on
  Math Function1 : Math  Operator=square  SaturateOnIntegerOverflow=on
  Math Function2 : Math  Operator=square  SaturateOnIntegerOverflow=on
  Product{1..5} (5 alike) : Product
  Saturation Dynamic1 : simulink/Discontinuities/Saturation Dynamic  OutMin=0  OutMax=1000  OutDataTypeStr=Inherit: Same as second input  OutDataType=fixdt(1, 16)  OutScaling=2^-10  DoSatur=off
  Saturation Dynamic2 : simulink/Discontinuities/Saturation Dynamic  OutMin=0  OutMax=1000  OutDataTypeStr=Inherit: Same as second input  OutDataType=fixdt(1, 16)  OutScaling=2^-10  DoSatur=off
  Sqrt1 : Sqrt  SaturateOnIntegerOverflow=on
  Sqrt2 : Sqrt  SaturateOnIntegerOverflow=on
  Sum{,1,3..4} (4 alike) : Sum  Inputs=|++
  Sum2 : Sum  Inputs=+-
  Sum5 : Sum  Inputs=+-
  Switch1 : Switch  Threshold=1
  Switch2 : Switch  Threshold=1
  Trigonometric Function : Trigonometry  Operator=tan
  friction_coeff : Constant  Value=0.85
  Out1 : Outport
  Out2 : Outport  Port=2
  Out3 : Outport  Port=3
  Out4 : Outport  Port=4
  wires:
  Sum2/1 -> Product3/1
  In4/1 -> Divide2/1
  Divide2/1 -> Switch1/2, Product3/2, Sum2/2
  Product3/1 -> Switch1/3
  Constant3/1 -> Sum2/1
  Constant2/1 -> Switch1/1
  friction_coeff/1 -> Divide1/2, Divide2/3
  Sum1/1 -> Divide11/3, Divide14/4, Divide2/2
  Constant/1 -> Product4/2, Product1/2, Divide14/3
  Gain1/1 -> Divide2/4
  Constant4/1 -> Sum4/1
  Product2/1 -> Divide4/1, Divide11/1, Math Function1/1
  Sum3/1 -> Sqrt2/1
  Sqrt2/1 -> Gain2/1
  Gain2/1 -> Divide1/4
  In1/1 -> Sum4/2, Product4/1
  Math Function2/1 -> Sum3/1
  Sum5/1 -> Product5/1
  In5/1 -> Divide1/1
  Math Function1/1 -> Sum3/2, Sum/1
  "Cornering_stiffness_r          "/1 -> Product2/1
  Switch1/1 -> Divide11/2, Divide14/1
  Divide1/1 -> Switch2/2, Sum5/2, Product5/2
  Constant6/1 -> Sum5/1
  In3/1 -> Divide14/2, Sum1/1, Product1/1
  Product1/1 -> Math Function/1
  Trigonometric Function/1 -> Product2/2
  Sum/1 -> Sqrt1/1
  Sqrt1/1 -> Gain1/1
  Constant1/1 -> Sum1/2
  In2/1 -> Trigonometric Function/1
  Math Function/1 -> Sum/2
  Constant5/1 -> Switch2/1
  Product4/1 -> Divide3/1, Math Function2/1
  Product5/1 -> Switch2/3
  Switch2/1 -> Divide4/2, Divide3/2
  Sum4/1 -> Divide4/3, Divide3/3, Divide1/3
  Divide11/1 -> Out2/1
  Divide4/1 -> Out3/1
  Saturation Dynamic1/1 -> Out1/1
  Divide14/1 -> Saturation Dynamic1/2
  Constant9/1 -> Saturation Dynamic1/1
  Constant10/1 -> Saturation Dynamic1/3
  Saturation Dynamic2/1 -> Out4/1
  Divide3/1 -> Saturation Dynamic2/2
  Constant11/1 -> Saturation Dynamic2/1
  Constant12/1 -> Saturation Dynamic2/3
